simulink model "simulink_model_closed_loop"  (R2013a)
settings: Solver=ode45  SolverMode=SingleTasking  StartTime=0.0  StopTime=1  RelTol=1e-3
values from neighbouring files (symbols this model uses):
  N = 40    [extensive_example_ocp.m]    (also in minimal_example_closed_loop.m = 20; minimal_example_ocp.m = 20)
  nu = model.nu    [extensive_example_ocp.m]    (also in minimal_example_closed_loop.m; minimal_example_ocp.m; minimal_example_sim.m)
  ny = nu+nx    [extensive_example_ocp.m]    (also in minimal_example_ocp.m = size(model.cost_expr_y, 1))
  ny_e = nx    [extensive_example_ocp.m]    (also in minimal_example_ocp.m = size(model.cost_expr_y_e, 1))
  U_max = 80    [minimal_example_closed_loop.m]    (also in minimal_example_ocp.m)
  x0 = [0; pi; 0; 0]    [extensive_example_ocp.m]    (also in minimal_example_closed_loop.m = x_sim(:,i); minimal_example_ocp.m; minimal_example_sim.m = [0; 1e-1; 0; 0])
settings Model: CovMetricSettings=dwe  CovHtmlReporting=off  covSaveCumulativeToWorkspaceVar=off  CovSaveSingleToWorkspaceVar=off  CovExternalEMLEnable=on  Creator=oj  LastModifiedBy=sandmann
settings DataIOCC: LimitDataPoints=off  SaveFormat=StructureWithTime  ReturnWorkspaceOutputs=on
settings DebuggingCC: UnderspecifiedInitializationDetection=Simplified  MergeDetectMultiDrivingBlocksExec=error  SolverPrmCheckMsg=none  FrameProcessingCompatibilityMsg=error  StateNameClashWarn=none  SFUnexpectedBacktrackingDiag=error  SFNoUnconditionalDefaultTransitionDiag=error
settings HardwareCC: ProdBitPerPointer=64  ProdLargestAtomicFloat=Float  ProdIntDivRoundTo=Zero  ProdEndianess=LittleEndian  ProdHWDeviceType=Specified
settings ModelReferenceCC: PropagateSignalLabelsOutOfModel=on
settings SFSimCC: SimUseLocalCustomCode=on
settings RTWCC: RTWUseLocalCustomCode=on
settings GRTTargetCC: CodeReplacementLibrary=C99 (ISO)

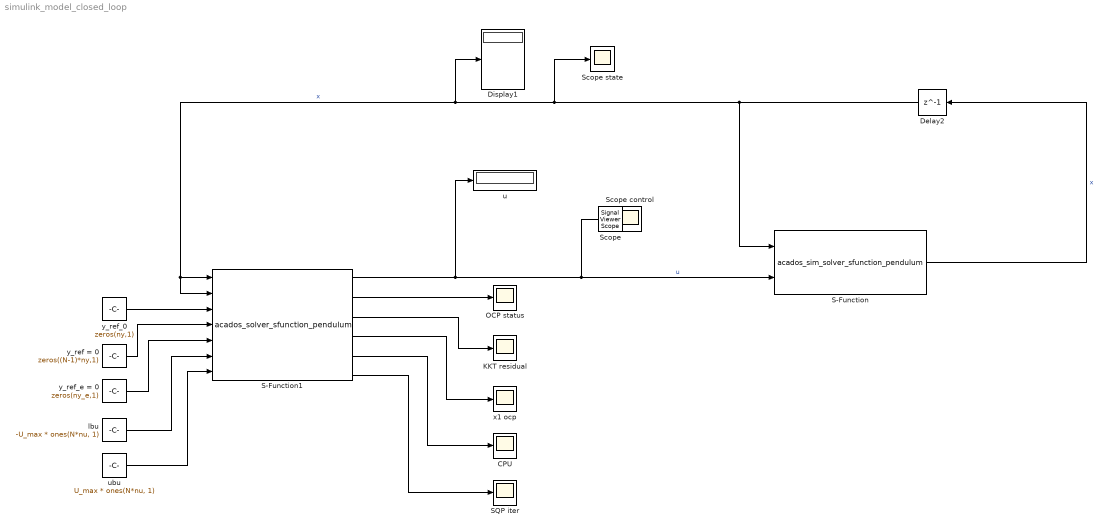
== system simulink_model_closed_loop ==
  CPU : Scope
      settings: Description=status  TimeRange=auto  MaxDataPoints=5000  SaveToWorkspace=off  SaveName=ScopeData3  YMin=-10  YMax=10  SampleTime=-1
  Delay2 : Delay  DelayLength=1  InitialCondition=x0
  Display1 : Display
  KKT residual : Scope
      settings: Description=status  TimeRange=auto  MaxDataPoints=5000  SaveToWorkspace=off  YMin=-0.000003  YMax=0.000031  SampleTime=-1
  OCP status : Scope
      settings: Description=status  TimeRange=auto  MaxDataPoints=5000  SaveToWorkspace=off  SaveName=ScopeData  YMin=-0.25  YMax=2.25  SampleTime=-1
  S-Function : S-Function  FunctionName=acados_sim_solver_sfunction_pendulum  SFunctionDeploymentMode=off  EnableBusSupport=off
  S-Function1 : S-Function  FunctionName=acados_solver_sfunction_pendulum  SFunctionDeploymentMode=off  EnableBusSupport=off
  SQP iter : Scope
      settings: Description=status  TimeRange=auto  MaxDataPoints=5000  SaveToWorkspace=off  YMin=-10  YMax=10  SampleTime=-1
  Scope control : Scope
      settings: TimeRange=auto  MaxDataPoints=5000  SaveToWorkspace=off  YMin=-100.00000  YMax=100.00000  SampleTime=-1
  Scope state : Scope
      settings: TimeRange=auto  MaxDataPoints=5000  SaveToWorkspace=off  YMin=-13.79726  YMax=10.28583  SampleTime=-1
  lbu : Constant  Value=-U_max * ones(N*nu, 1)
  u : Display
  ubu : Constant  Value=U_max * ones(N*nu, 1)
  x1 ocp : Scope
      settings: Description=status  TimeRange=auto  MaxDataPoints=5000  SaveToWorkspace=off  SaveName=ScopeData2  YMin=-0.0000000002  YMax=0.0000000026  SampleTime=-1
  y_ref = 0 : Constant  Value=zeros((N-1)*ny,1)
  y_ref_0 : Constant  Value=zeros(ny,1)
  y_ref_e = 0 : Constant  Value=zeros(ny_e,1)
  Scope : SignalViewerScope  IOType=viewer  SampleTime=-1  ZoomMode=on
      settings: TimeRange=auto  TickLabels=OneTimeTick  MaxDataPoints=5000  SaveToWorkspace=off  YMin=-13.79726  YMax=10.28583  SampleInput=off  DataFormat=StructureWithTime
  wires:
  S-Function/1 -> Delay2/1  "x"
  S-Function1/2 -> OCP status/1
  S-Function1/3 -> KKT residual/1
  S-Function1/4 -> x1 ocp/1
  S-Function1/5 -> CPU/1
  lbu/1 -> S-Function1/6
  S-Function1/1 -> u/1, Scope control/1, S-Function/2  "u"
  Delay2/1 -> S-Function/1, S-Function1/2, S-Function1/1, Display1/1, Scope state/1  "x"
  S-Function1/6 -> SQP iter/1
  ubu/1 -> S-Function1/7
  y_ref_e = 0/1 -> S-Function1/5
  y_ref = 0/1 -> S-Function1/4
  y_ref_0/1 -> S-Function1/3
